simulink model "Ex3"  (R2013a)
settings: Solver=ode45  StartTime=0.0  StopTime=15  RelTol=1e-3
settings Model: Creator=Sudip Sinha  LastModifiedBy=Sudip Sinha

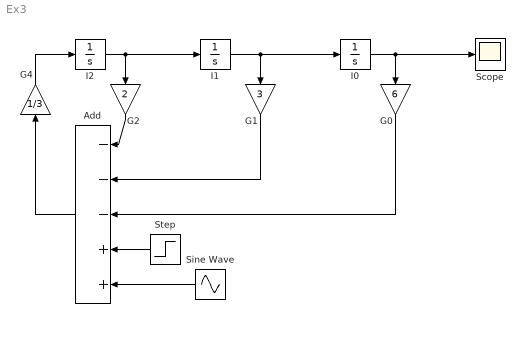
== system Ex3 ==
  Add : Sum  Inputs=---++
  G0 : Gain  Gain=6
  G1 : Gain  Gain=3
  G2 : Gain  Gain=2
  G4 : Gain  Gain=1/3
  I0 : Integrator  InitialCondition=1
  I1 : Integrator  InitialCondition=2
  I2 : Integrator  InitialCondition=-3
  Scope : Scope
  Sine Wave : Sin  Frequency=2  Phase=pi/2  SampleTime=0
  Step : Step  After=3  SampleTime=0
  wires:
  I2/1 -> I1/1, G2/1
  I1/1 -> I0/1, G1/1
  I0/1 -> Scope/1, G0/1
  G0/1 -> Add/3
  G1/1 -> Add/2
  G2/1 -> Add/1
  Step/1 -> Add/4
  Sine Wave/1 -> Add/5
  Add/1 -> G4/1
  G4/1 -> I2/1
